simulink model "controller_arduino"  (R2024b)
settings: Solver=FixedStepAuto  StartTime=0.0  StopTime=10.0  RelTol=1e-3
undefined symbols (not defined in the file): TransmissionState
libraries: arduinolib x5
settings Model: Creator=WxxGr  LastModifiedBy=WxxGr

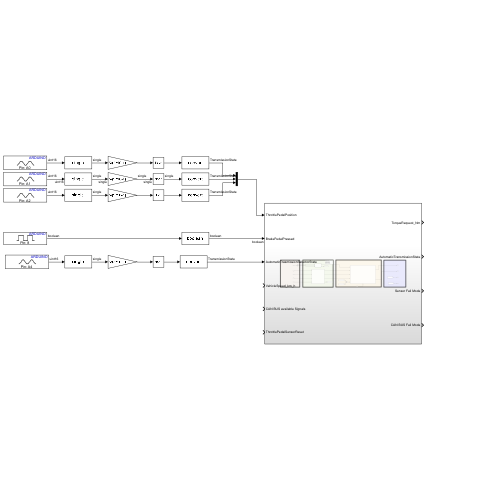
[thumbnail: Simulink's stored preview of the top-level diagram]
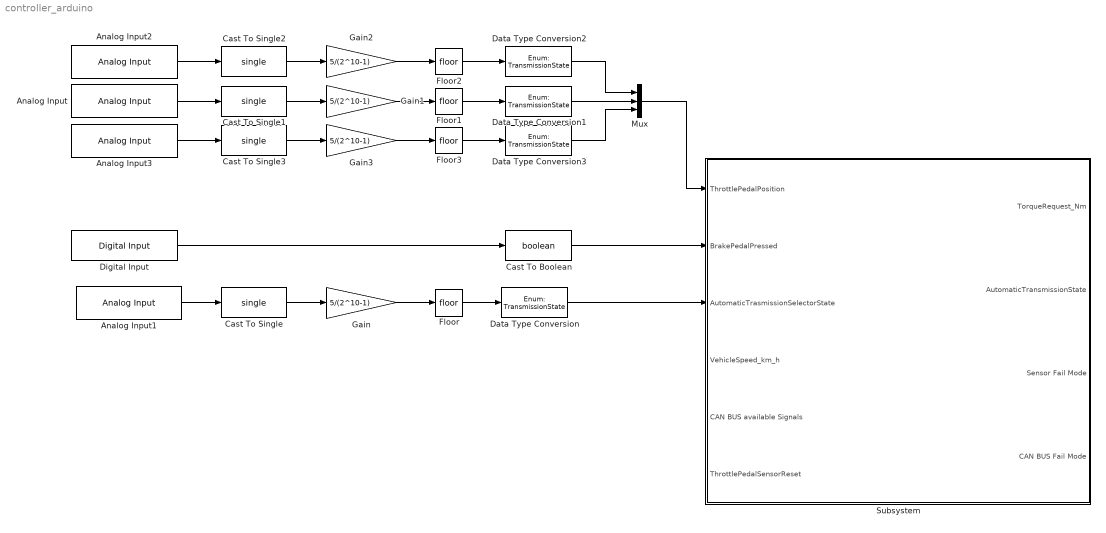
== system controller_arduino ==
  Analog Input : arduinolib/Analog Input  pinNumber=1  ReadResultsOnly=off  ConversionTriggerSource=Software  ExternalTriggerType=uint32( 0 )  OutputDataType=uint16  EnableConversionCompleteNotify=off  EnableOuputStatus=off  SampleTime=-1  blockPlatform=arduino
      settings: SourceProductName=Common
  Analog Input1 : arduinolib/Analog Input  pinNumber=4  ReadResultsOnly=off  ConversionTriggerSource=Software  ExternalTriggerType=uint32( 0 )  OutputDataType=uint16  EnableConversionCompleteNotify=off  EnableOuputStatus=off  SampleTime=-1  blockPlatform=arduino
      settings: SourceProductName=Common
  Analog Input2 : arduinolib/Analog Input  pinNumber=0  ReadResultsOnly=off  ConversionTriggerSource=Software  ExternalTriggerType=uint32( 0 )  OutputDataType=uint16  EnableConversionCompleteNotify=off  EnableOuputStatus=off  SampleTime=-1  blockPlatform=arduino
      settings: SourceProductName=Common
  Analog Input3 : arduinolib/Analog Input  pinNumber=2  ReadResultsOnly=off  ConversionTriggerSource=Software  ExternalTriggerType=uint32( 0 )  OutputDataType=uint16  EnableConversionCompleteNotify=off  EnableOuputStatus=off  SampleTime=-1  blockPlatform=arduino
      settings: SourceProductName=Common
  Cast To Boolean : DataTypeConversion  OutDataTypeStr=boolean  SaturateOnIntegerOverflow=off  RndMeth=Floor
  Cast To Single{,1..3} (4 alike) : DataTypeConversion  OutDataTypeStr=single  SaturateOnIntegerOverflow=off  RndMeth=Floor
  Data Type Conversion{,1..3} (4 alike) : DataTypeConversion  OutDataTypeStr=Enum: TransmissionState  SaturateOnIntegerOverflow=off  RndMeth=Floor
  Digital Input : arduinolib/Digital Input  pinNumber=8  mode=Default  Direction=input  SampleTime=0.1  blockPlatform=arduino
      settings: SourceProductName=Common
  Floor{,1..3} (4 alike) : Rounding
  Gain{,1..3} (4 alike) : Gain  Gain=5/(2^10-1)
  Mux : Mux  Inputs=3
  Subsystem : Subsystem
  wires:
  Digital Input/1 -> Cast To Boolean/1
  Analog Input1/1 -> Cast To Single/1
  Cast To Single/1 -> Gain/1
  Gain/1 -> Floor/1
  Floor/1 -> Data Type Conversion/1
  Data Type Conversion/1 -> Subsystem/3(AutomaticTrasmissionSelectorState)
  Cast To Boolean/1 -> Subsystem/2(BrakePedalPressed)
  Analog Input/1 -> Cast To Single1/1
  Cast To Single1/1 -> Gain1/1
  Floor1/1 -> Data Type Conversion1/1
  Gain1/1 -> Floor1/1
  Data Type Conversion1/1 -> Mux/2
  Mux/1 -> Subsystem/1(ThrottlePedalPosition)
  Floor2/1 -> Data Type Conversion2/1
  Analog Input2/1 -> Cast To Single2/1
  Gain2/1 -> Floor2/1
  Cast To Single2/1 -> Gain2/1
  Data Type Conversion2/1 -> Mux/1
  Floor3/1 -> Data Type Conversion3/1
  Analog Input3/1 -> Cast To Single3/1
  Gain3/1 -> Floor3/1
  Cast To Single3/1 -> Gain3/1
  Data Type Conversion3/1 -> Mux/3

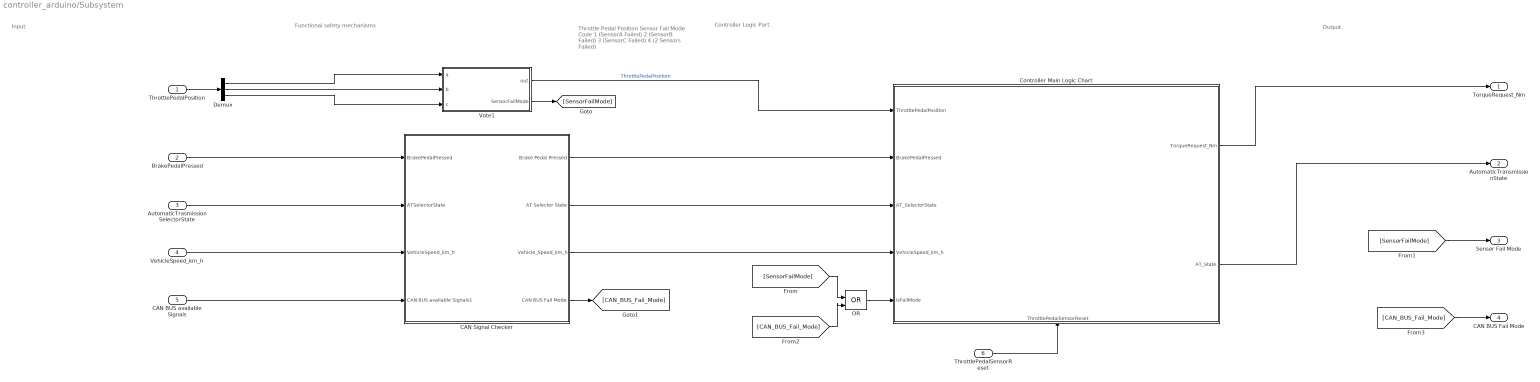
== system controller_arduino/Subsystem ==
  note: Output
  note: Functional safety mechanisms
  note: Throttle Pedal Position Sensor
      | Fail Mode Code
      | 1 (SensorA Failed)
      | 2 (SensorB Failed)
      | 3 (SensorC Failed)
      | 4 (2 Sensors Failed)
  note: Input
  note: Controller Logic Part
  ThrottlePedalPosition : Inport
  BrakePedalPressed : Inport  Port=2  OutDataTypeStr=boolean
  AutomaticTrasmissionSelectorState : Inport  Port=3
  VehicleSpeed_km_h : Inport  Port=4  OutDataTypeStr=single  Unit=km/h
  CAN BUS available Signals : Inport  Port=5  OutDataTypeStr=boolean  Unit=km/h
  ThrottlePedalSensorReset : Inport  Port=6  OutDataTypeStr=boolean  Unit=km/h
  CAN Signal Checker : Subsystem
  "Controller Main Logic Chart " : Stateflow chart  TreatAsAtomicUnit=on
      settings: PortSchema="{\"entries\":[{\"content\":{\"sides\":[{\"content\":{\"connectorIds\":[\"In2\",\"In1\",\"In3\",\"In4\",\"In5\"]},\"type\":\"ConnectorPlacement.EquallySpacedRectSide\",\"uuid\":\"c1d5eae4-5946-42bc-859d-819865b27d40\"},{\"content\":{\"connectorIds\":[\"Out2\",\"Out1\"],\"side\":\"RIGHT\"},\"type\":\"ConnectorPlacement.EquallySpacedRectSide\",\"uuid\":\"cb8f30de-ae1c-4452-b388-6390164ac5c5\"},{\"content\":{\"side\":\"TOP\"},\"type\":\"ConnectorPlacement.EquallySpacedRectSide\",\"uuid\":\"d645f778-68a3-4694-8aeb-1853997d5a7f\"},{\"content\":{\"connectorIds\":[\"In6\"],\"side\":\"BOTTOM\"},\"type\":\"ConnectorPlacement.EquallySpacedRectSide\",\"uuid\":\"52e35704-7e66-4a7d-b4fe-753f82e5d6b3\"}]},\"type\":\"ConnectorPlacement.EquallySpacedConnector\",\"uuid\":\"d99be1ad-e6ff-4f7e-a1bd-fa4b5370c86d\"}],\"packageUris\":[\"http://schema.mathworks.com/mf0/Connector/R2020b\"],\"version\":\"1.0\"}"
  Demux : Demux  Outputs=3
  OR : Logic  Operator=OR  IconShape=distinctive  AllPortsSameDT=off  OutDataTypeStr=boolean
  Vote1 : Stateflow chart  TreatAsAtomicUnit=on
  TorqueRequest_Nm : Outport  OutDataTypeStr=single  Unit=N*m
  AutomaticTransmissionState : Outport  Port=2  OutDataTypeStr=Enum: TransmissionState
  Sensor Fail Mode : Outport  Port=3  OutDataTypeStr=int8
  CAN BUS Fail Mode : Outport  Port=4  OutDataTypeStr=int8
  wires:
  VehicleSpeed_km_h/1 -> CAN Signal Checker/3(VehicleSpeed_km_h)
  Demux/1 -> Vote1/1(a)
  [SensorFailMode] -> OR/1
  AutomaticTrasmissionSelectorState/1 -> CAN Signal Checker/2(ATSelectorState)
  [CAN_BUS_Fail_Mode] -> CAN BUS Fail Mode/1
  [CAN_BUS_Fail_Mode] -> OR/2
  CAN BUS available Signals/1 -> CAN Signal Checker/4(CAN BUS available Signals1)
  CAN Signal Checker/4(CAN BUS Fail Mode) -> [CAN_BUS_Fail_Mode]
  Vote1/2(SensorFailMode) -> [SensorFailMode]
  CAN Signal Checker/3(Vehicle_Speed_km_h) -> "Controller Main Logic Chart "/4(VehicleSpeed_km_h)
  CAN Signal Checker/1(Brake Pedal Pressed) -> "Controller Main Logic Chart "/1(BrakePedalPressed)
  Demux/3 -> Vote1/3(c)
  Vote1/1(out) -> "Controller Main Logic Chart "/2(ThrottlePedalPosition)  "ThrottlePedalPosition"
  [SensorFailMode] -> Sensor Fail Mode/1
  BrakePedalPressed/1 -> CAN Signal Checker/1(BrakePedalPressed)
  "Controller Main Logic Chart "/1(AT_State) -> AutomaticTransmissionState/1
  "Controller Main Logic Chart "/2(TorqueRequest_Nm) -> TorqueRequest_Nm/1
  ThrottlePedalSensorReset/1 -> "Controller Main Logic Chart "/6(ThrottlePedalSensorReset)
  CAN Signal Checker/2(AT Selector State) -> "Controller Main Logic Chart "/3(AT_SelectorState)
  OR/1 -> "Controller Main Logic Chart "/5(isFailMode)
  ThrottlePedalPosition/1 -> Demux/1
  Demux/2 -> Vote1/2(b)

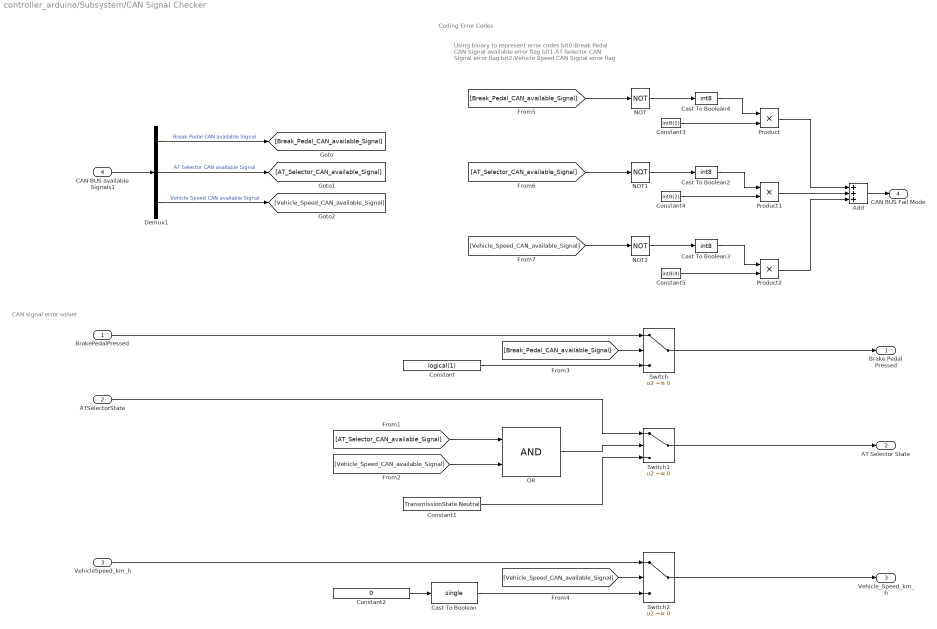
== system controller_arduino/Subsystem/CAN Signal Checker ==
  note: CAN signal error solver
  note: Coding Error Codes
  note: Using binary to represent error codes
      | bit0:Break Pedal CAN Signal available error flag
      | bit1:AT Selector CAN Signal error flag
      | bit2:Vehicle Speed CAN Signal error flag
  BrakePedalPressed : Inport
  ATSelectorState : Inport  Port=2
  VehicleSpeed_km_h : Inport  Port=3
  CAN BUS available Signals1 : Inport  Port=4
  Add : Sum  Inputs=+++
  Cast To Boolean : DataTypeConversion  OutDataTypeStr=single  SaturateOnIntegerOverflow=off  RndMeth=Floor
  Cast To Boolean2 : DataTypeConversion  OutDataTypeStr=int8  SaturateOnIntegerOverflow=off  RndMeth=Floor
  Cast To Boolean3 : DataTypeConversion  OutDataTypeStr=int8  SaturateOnIntegerOverflow=off  RndMeth=Floor
  Cast To Boolean4 : DataTypeConversion  OutDataTypeStr=int8  SaturateOnIntegerOverflow=off  RndMeth=Floor
  Constant : Constant  Value=logical(1)
  Constant1 : Constant  Value=TransmissionState.Neutral
  Constant2 : Constant  Value=0
  Constant3 : Constant  Value=int8(1)
  Constant4 : Constant  Value=int8(2)
  Constant5 : Constant  Value=int8(4)
  Demux1 : Demux  Outputs=3
  NOT : Logic  Operator=NOT  IconShape=distinctive  AllPortsSameDT=off  OutDataTypeStr=boolean
  NOT1 : Logic  Operator=NOT  IconShape=distinctive  AllPortsSameDT=off  OutDataTypeStr=boolean
  NOT2 : Logic  Operator=NOT  IconShape=distinctive  AllPortsSameDT=off  OutDataTypeStr=boolean
  OR : Logic  AllPortsSameDT=off  OutDataTypeStr=boolean
  Product : Product  OutDataTypeStr=int8
  Product1 : Product  OutDataTypeStr=int8
  Product2 : Product  OutDataTypeStr=int8
  Switch : Switch  Criteria=u2 ~= 0  SaturateOnIntegerOverflow=off  InputSameDT=off
  Switch1 : Switch  Criteria=u2 ~= 0  SaturateOnIntegerOverflow=off  InputSameDT=off
  Switch2 : Switch  Criteria=u2 ~= 0  SaturateOnIntegerOverflow=off  InputSameDT=off
  Brake Pedal Pressed : Outport
  AT Selector State : Outport  Port=2
  Vehicle_Speed_km_h : Outport  Port=3  OutDataTypeStr=single
  CAN BUS Fail Mode : Outport  Port=4
  wires:
  Switch/1 -> Brake Pedal Pressed/1
  Constant/1 -> Switch/3
  BrakePedalPressed/1 -> Switch/1
  Switch1/1 -> AT Selector State/1
  ATSelectorState/1 -> Switch1/1
  Constant1/1 -> Switch1/3
  OR/1 -> Switch1/2
  Switch2/1 -> Vehicle_Speed_km_h/1
  VehicleSpeed_km_h/1 -> Switch2/1
  Constant2/1 -> Cast To Boolean/1
  CAN BUS available Signals1/1 -> Demux1/1
  Demux1/2 -> [AT_Selector_CAN_available_Signal]  "AT Selector CAN available Signal"
  Demux1/1 -> [Break_Pedal_CAN_available_Signal]  "Break Pedal CAN available Signal"
  Demux1/3 -> [Vehicle_Speed_CAN_available_Signal]  "Vehicle Speed CAN available Signal"
  [AT_Selector_CAN_available_Signal] -> OR/1
  [Vehicle_Speed_CAN_available_Signal] -> OR/2
  [Break_Pedal_CAN_available_Signal] -> Switch/2
  [Vehicle_Speed_CAN_available_Signal] -> Switch2/2
  Constant3/1 -> Product/2
  [Break_Pedal_CAN_available_Signal] -> NOT/1
  Constant4/1 -> Product1/2
  [AT_Selector_CAN_available_Signal] -> NOT1/1
  Constant5/1 -> Product2/2
  [Vehicle_Speed_CAN_available_Signal] -> NOT2/1
  Product/1 -> Add/1
  Product1/1 -> Add/2
  Product2/1 -> Add/3
  Add/1 -> CAN BUS Fail Mode/1
  Cast To Boolean/1 -> Switch2/3
  Cast To Boolean4/1 -> Product/1
  Cast To Boolean2/1 -> Product1/1
  Cast To Boolean3/1 -> Product2/1
  NOT/1 -> Cast To Boolean4/1
  NOT1/1 -> Cast To Boolean2/1
  NOT2/1 -> Cast To Boolean3/1

== stateflow chart controller_arduino/Subsystem/Vote1 ==
  note: When the absolute differences between any two of the three sensors — sensor a , sensor b , and sensor c — are all within 0.001, and the outputs of all three sensors are within the range [0, 1], then all three sensor readings are considered valid.
      | Output: out = (a + b + c) / 3
      | If any sensor has an absolute difference greater than 0.001 compared to the other two sensors, or its output is outside the range [0, 1], that sensor is considered invalid and ignored.
      | Output: out = (a + b) / 2 (where a and b are the remaining valid sensors)
      | If, at the previous time step, only two sensors were still considered valid, but now their absolute difference exceeds 0.001, or either of their outputs is outside the [0, 1] range, it is assumed that two sensors have failed and no reliable sensor data is available.
      | Output: out = 0
  state Normal
    du:
    abDiff = single(abs(a-b));
    acDiff = single(abs(a-c));
    bcDiff = single(abs(b-c));
    if   a<0 || a>1 || (abDiff>Torlance && acDiff>Torlance)  %%A failure
    out = (b+c)/2;
    SensorFailMode = 1;
    elseif b>1 || b<0 || abDiff>Torlance  %%B failure
    out = (a+c)/2;
    SensorFailMode = 2;
    elseif c>1 || c<0 || acDiff>Torlance %%C failure
    out = (a+b)/2;
    SensorFailMode = 3;
    else
    out = (a+b+c)/3;
    end
  note: EmergencyMode Code
      | 1 (SensorA Failed)
      | 2 (SensorB Failed)
      | 3 (SensorC Failed)
      | 4 (2 Sensors Failed)
  note: We assume that the throttle pedal angle sensor is calibrated to ±0.0005 error between [0 1]
      |
      | So the difference between any two throttle pedal angles should not be greater than 0.001
  state A_Failure
    en:
    out = (b+c)/2;
    du:
    bcDiff = abs(b-c);
    if bcDiff>Torlance||b>1||b<0||c>1||c<0
    SensorFailMode = 4;
    out = 0;
    else
    out = (b+c)/2;
    end
  state B_Failure
    en:
    out = (a+c)/2;
    du:
    acDiff = abs(a-c);
    if acDiff>Torlance||a>1||a<0||c>1||c<0
    SensorFailMode = 4;
    out = 0;
    else
    out = (a+c)/2;
    end
  state C_Failure
    en:
    out = (a+b)/2;
    du:
    abDiff = abs(a-b);
    if abDiff>Torlance||b>1||b<0||a>1||a<0
    SensorFailMode = 4;
    out = 0;
    else
    out = (a+b)/2;
    end
  state NO_Trust
    en:
    out = 0;
  note: //Fail
  (default) -> Normal
  Normal -> C_Failure [order 2] : [SensorFailMode == 3]
  Normal -> A_Failure [order 1] : [SensorFailMode == 1]
  Normal -> B_Failure [order 3] : [SensorFailMode == 2]
  A_Failure -> NO_Trust : [SensorFailMode == 4]
  B_Failure -> NO_Trust : [SensorFailMode == 4]
  C_Failure -> NO_Trust : [SensorFailMode == 4]
  NO_Trust -> NO_Trust
  data: out output single; a input single; b input single; SensorFailMode output int8 =0; c input single; abDiff local single =0; acDiff local single =0; bcDiff local single =0; Torlance local single =0.001

== stateflow chart controller_arduino/Subsystem/Controller Main Logic Chart  ==
  state NoFailureDetected
    state Park
      en:
      AT_State =TransmissionState.Park;
      du:
      TorqueRequest_Nm = 0;
    state Brake
      en:
      AT_State =TransmissionState.Brake;
      state BrakeNormalCondition
        state brakeAccle
          du:
          TorqueRequest_Nm = single(ThrottlePedalPosition-1/3)*1.5 * 80;
        state barkDecele
          du:
          TorqueRequest_Nm = -3*single(1/3-ThrottlePedalPosition) * 80;
        state brak0Velocity
          du:
          %Add a PI controller
          error = 0 - VehicleSpeed_km_h;
          sumError = sumError + error;
          TorqueRequest_Nm = error*30+sumError*2;
          ex:sumError = 0;
        (default) -> brakeAccle
        brakeAccle -> barkDecele : [ThrottlePedalPosition<=1/3]
        barkDecele -> brakeAccle [order 1] : [ThrottlePedalPosition>1/3]
        (junction 83) -> brakeAccle
        barkDecele -> brak0Velocity [order 2] : [VehicleSpeed_km_h <= 0.2]
        brak0Velocity -> (junction 83) : [ThrottlePedalPosition>1/3]
      state barkStop
        en:
        TorqueRequest_Nm = 0;
      barkStop -> BrakeNormalCondition : [BrakePedalPressed ~=1]
      BrakeNormalCondition -> barkStop : [BrakePedalPressed ==1]
      (default) -> barkStop
    state Drive
      en:
      AT_State =TransmissionState.Drive;
      state normalDrive
        du:
        TorqueRequest_Nm = single(ThrottlePedalPosition) * 80;
      state driveStop
        du:
        TorqueRequest_Nm = 0;
      NoFailureDetected.Drive.normalDrive -> NoFailureDetected.Drive.driveStop : [BrakePedalPressed ==1]
      NoFailureDetected.Drive.driveStop -> NoFailureDetected.Drive.normalDrive : [BrakePedalPressed~=1]
      (default) -> NoFailureDetected.Drive.driveStop
    state Neutral
      en:
      AT_State =TransmissionState.Neutral;
      du:
      TorqueRequest_Nm = 0;
    state Reverse
      en:
      AT_State =TransmissionState.Reverse;
      state normalReverse
        du:
        TorqueRequest_Nm = -single(ThrottlePedalPosition) * 40;
      state reverseStop
        du:
        TorqueRequest_Nm = 0;
      NoFailureDetected.Reverse.normalReverse -> NoFailureDetected.Reverse.reverseStop : [BrakePedalPressed == 1]
      NoFailureDetected.Reverse.reverseStop -> NoFailureDetected.Reverse.normalReverse : [BrakePedalPressed ~= 1]
      (default) -> NoFailureDetected.Reverse.reverseStop
    (default) -> NoFailureDetected.Park
    NoFailureDetected.Park -> NoFailureDetected.Neutral : [BrakePedalPressed == 1 &&...
        | AT_SelectorState ~= TransmissionState.Park ]
    NoFailureDetected.Neutral -> NoFailureDetected.Park [order 1] : [VehicleSpeed_km_h<5 &&...
        | VehicleSpeed_km_h>-5 &&...
        | BrakePedalPressed == 1 &&...
        | AT_SelectorState == TransmissionState.Park ]
    NoFailureDetected.Drive -> NoFailureDetected.Neutral [order 1] : [AT_SelectorState == TransmissionState.Neutral]
    Brake -> NoFailureDetected.Drive : [AT_SelectorState ==TransmissionState.Drive||...
        | AT_SelectorState ==TransmissionState.Neutral]
    NoFailureDetected.Neutral -> NoFailureDetected.Reverse [order 2] : [VehicleSpeed_km_h < 5 &&...
        | BrakePedalPressed == 1 &&...
        | AT_SelectorState == TransmissionState.Reverse]
    NoFailureDetected.Neutral -> NoFailureDetected.Drive [order 3] : [VehicleSpeed_km_h>-5 &&...
        | BrakePedalPressed == 1 &&...
        | (AT_SelectorState ==TransmissionState.Drive ||...
        | AT_SelectorState ==TransmissionState.Brake) ]
    NoFailureDetected.Reverse -> NoFailureDetected.Neutral : [AT_SelectorState  ~= TransmissionState.Reverse]
    NoFailureDetected.Drive -> Brake [order 2] : [ThrottlePedalPosition>1/3 &&...
        | AT_SelectorState ==TransmissionState.Brake]
  state LimpMode %When any sensor/CAN signal failure, enter this protect mode (with power constraints)
    state Park
      en:
      AT_State = TransmissionState.Park;
      du:
      TorqueRequest_Nm = 0;
    state Drive
      en:
      AT_State =TransmissionState.Drive;
      state normalDrive
        du:
        if VehicleSpeed_km_h < 20
        TorqueRequest_Nm = single(ThrottlePedalPosition) * 80 / 10;
        else
        TorqueRequest_Nm = 0;
        end
      state driveStop
        du:
        TorqueRequest_Nm = 0;
      LimpMode.Drive.normalDrive -> LimpMode.Drive.driveStop : [BrakePedalPressed ==1]
      LimpMode.Drive.driveStop -> LimpMode.Drive.normalDrive : [BrakePedalPressed~=1]
      (default) -> LimpMode.Drive.driveStop
    state Neutral
      en:
      AT_State =TransmissionState.Neutral;
      du:
      TorqueRequest_Nm = 0;
    state Reverse
      en:
      AT_State =TransmissionState.Reverse;
      state normalReverse
        du:
        TorqueRequest_Nm = -8*single(ThrottlePedalPosition) * 60/12/10;
      state reverseStop
        du:
        TorqueRequest_Nm = 0;
      LimpMode.Reverse.normalReverse -> LimpMode.Reverse.reverseStop : [BrakePedalPressed == 1]
      LimpMode.Reverse.reverseStop -> LimpMode.Reverse.normalReverse : [BrakePedalPressed ~= 1]
      (default) -> LimpMode.Reverse.reverseStop
    (default) -> (junction 161)
    (junction 161) -> (junction 167) [order 4] : [lastTimeMode == TransmissionState.Reverse]
    (junction 161) -> LimpMode.Park [order 5]
    (junction 161) -> LimpMode.Drive [order 3] : [lastTimeMode == TransmissionState.Brake]
    (junction 161) -> LimpMode.Neutral [order 1] : [lastTimeMode == TransmissionState.Neutral]
    (junction 161) -> LimpMode.Drive [order 2] : [lastTimeMode == TransmissionState.Drive]
    (junction 167) -> LimpMode.Reverse
    LimpMode.Park -> LimpMode.Neutral : [BrakePedalPressed == 1 &&...
        | AT_SelectorState ~= TransmissionState.Park ]
    LimpMode.Neutral -> LimpMode.Park [order 1] : [VehicleSpeed_km_h<5 &&...
        | VehicleSpeed_km_h>-5 &&...
        | BrakePedalPressed == 1 &&...
        | AT_SelectorState == TransmissionState.Park ]
    LimpMode.Drive -> LimpMode.Neutral : [AT_SelectorState == TransmissionState.Neutral]
    LimpMode.Neutral -> LimpMode.Reverse [order 2] : [VehicleSpeed_km_h < 5 &&...
        | BrakePedalPressed == 1 &&...
        | AT_SelectorState == TransmissionState.Reverse]
    LimpMode.Neutral -> LimpMode.Drive [order 3] : [VehicleSpeed_km_h> -5 &&...
        | BrakePedalPressed == 1 &&...
        | (AT_SelectorState ==TransmissionState.Drive ||...
        | AT_SelectorState ==TransmissionState.Brake) ]
    LimpMode.Reverse -> LimpMode.Neutral : [AT_SelectorState  ~= TransmissionState.Reverse]
  (default) -> NoFailureDetected
  NoFailureDetected -> LimpMode %When any sensor/CAN signal failure, enter this protect mode (with power constraints) : [isFailMode ~= 0]
      | {lastTimeMode = AT_State;}
  LimpMode %When any sensor/CAN signal failure, enter this protect mode (with power constraints) -> NoFailureDetected : [ThrottlePedalSensorReset == 1]
  data: AT_State output; BrakePedalPressed input; ThrottlePedalPosition input; AT_SelectorState input; VehicleSpeed_km_h input; TorqueRequest_Nm output single; sumError local single =0; error local; isFailMode input boolean; ThrottlePedalSensorReset input boolean; lastTimeMode local
